simulink model "Y6_sim"  (R2024b)
settings: Solver=VariableStepAuto  StartTime=0.0  StopTime=580  RelTol=1e-3
values from neighbouring files (symbols this model uses):
  states0 = [42;0;0;0;0;0;0;0;0;0;0;0]    [Y6_params.m]
  timepoints = [0,30,55,80,105,130,165,190,215,240,265,300,325,350,375,400,435,460,485,510,535,570]    [Y6_params.m]
  waypoints = [42  ,42  ,42   ,42   ,42   ,42   ,31   ,31   ,31   ,31   ,31   ,20   ,20   ,20   ,20   ,20   ,9    ,9    ,9    ,9    ,9    ,9 ... (first row only)    [Y6_params.m]
libraries: shareduavrstlib x1, simulink x1, uavutilslib x1
settings Model: Creator=efymc10  LastModifiedBy=louis
settings SolverCC: ZeroCrossAlgorithm=Adaptive
settings DebuggingCC: IgnoredZcDiagnostic=none

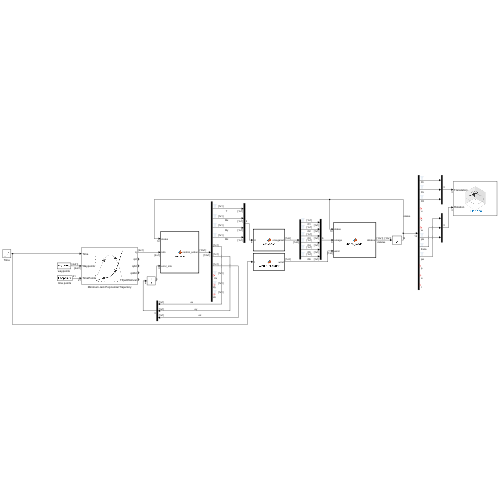
[thumbnail: Simulink's stored preview of the top-level diagram]
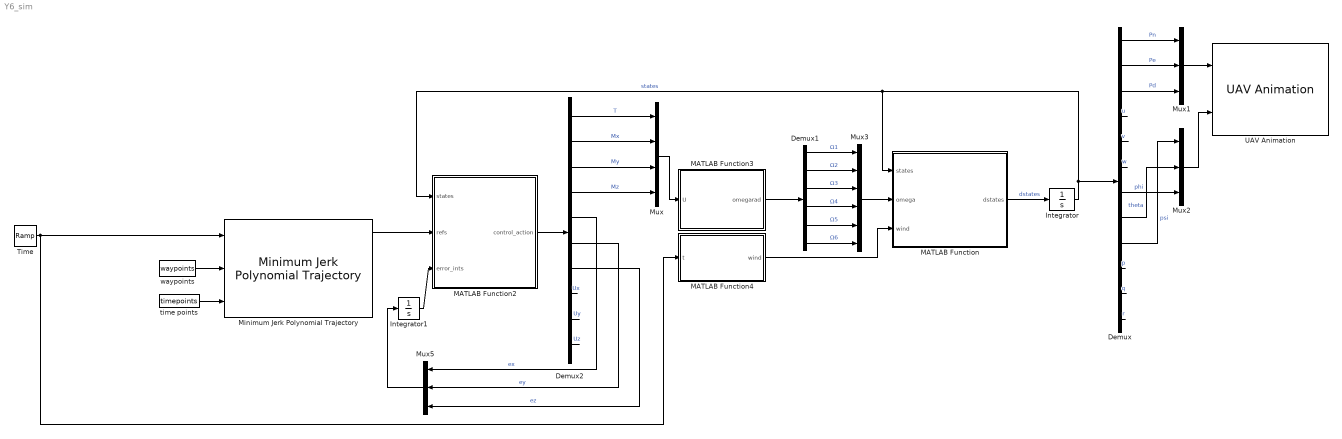
== system Y6_sim ==
  Demux : Demux  Outputs=12
  Demux1 : Demux  Outputs=6
  Demux2 : Demux  Outputs=10
  Integrator : Integrator  InitialCondition=states0
  Integrator1 : Integrator
  MATLAB Function : MATLAB Function  TreatAsAtomicUnit=on
  MATLAB Function2 : MATLAB Function  TreatAsAtomicUnit=on
  MATLAB Function3 : MATLAB Function  TreatAsAtomicUnit=on
  MATLAB Function4 : MATLAB Function  TreatAsAtomicUnit=on
  Minimum Jerk Polynomial Trajectory : shareduavrstlib/Minimum Jerk Polynomial Trajectory  ShowBCInputPort=off  ShowPolynomialCoefs=off  ShowStatusOutputPort=off  TimeAllocation=off  TimeWeight=100  MinSegmentTime=0.1  MaxSegmentTime=1  MaxIteration=1500  MaxTime=10  SimulateUsing=Interpreted execution
      settings: LibrarySourceBlock=uavalgslib/Minimum Jerk Polynomial Trajectory
  Mux : Mux
  Mux1 : Mux  Inputs=3
  Mux2 : Mux  Inputs=3
  Mux3 : Mux  Inputs=6
  Mux5 : Mux  Inputs=3
  Time : simulink/Sources/Ramp  slope=1  start=0  InitialOutput=0
  UAV Animation : uavutilslib/UAV Animation  NumUAV=1  DynamicUAVConfig=off  UAVType=Multirotor  UAVSize=1  UAVColor=[1 0 0]  UAVTrajectoryAlpha=1  InertialZDirection=Down  RotationFormat=Euler ZYX  DrawMarkers=off  SampleTime=0.01
  time points : Constant  Value=timepoints
  waypoints : Constant  Value=waypoints
  wires:
  Integrator/1 -> MATLAB Function2/1(states), MATLAB Function/1(states), Demux/1  "states"
  MATLAB Function/1(dstates) -> Integrator/1  "dstates"
  Demux/1 -> Mux1/1  "Pn"
  Demux/2 -> Mux1/2  "Pe"
  Demux/9 -> Mux2/1  "psi"
  Demux/7 -> Mux2/3  "phi"
  Demux/3 -> Mux1/3  "Pd"
  Demux/8 -> Mux2/2  "theta"
  Mux1/1 -> UAV Animation/1
  Mux2/1 -> UAV Animation/2
  time points/1 -> Minimum Jerk Polynomial Trajectory/3
  Minimum Jerk Polynomial Trajectory/1 -> MATLAB Function2/2(refs)
  Time/1 -> MATLAB Function4/1(t), Minimum Jerk Polynomial Trajectory/1
  MATLAB Function4/1(wind) -> MATLAB Function/3(wind)
  MATLAB Function2/1(control_action) -> Demux2/1
  Demux2/1 -> Mux/1  "T"
  Demux2/2 -> Mux/2  "Mx"
  Demux2/3 -> Mux/3  "My"
  Demux2/4 -> Mux/4  "Mz"
  Demux2/5 -> Mux5/1  "ex"
  Demux2/6 -> Mux5/2  "ey"
  Demux2/7 -> Mux5/3  "ez"
  Mux5/1 -> Integrator1/1
  Integrator1/1 -> MATLAB Function2/3(error_ints)
  Demux2/8 -> ?  "Ux"
  Demux2/9 -> ?  "Uy"
  Demux2/10 -> ?  "Uz"
  Demux/4 -> ?  "u"
  Demux/5 -> ?  "v"
  Demux/6 -> ?  "w"
  Demux/10 -> ?  "p"
  Demux/11 -> ?  "q"
  Demux/12 -> ?  "r"
  Demux1/1 -> Mux3/1  "Ω1"
  Demux1/2 -> Mux3/2  "Ω2"
  Demux1/3 -> Mux3/3  "Ω3"
  Demux1/4 -> Mux3/4  "Ω4"
  Demux1/5 -> Mux3/5  "Ω5"
  Demux1/6 -> Mux3/6  "Ω6"
  MATLAB Function3/1(omegarad) -> Demux1/1
  Mux3/1 -> MATLAB Function/2(omega)
  Mux/1 -> MATLAB Function3/1(U)
  waypoints/1 -> Minimum Jerk Polynomial Trajectory/2

== matlab function Y6_sim/MATLAB Function ==
  data: states input; dstates output; omega input; Y6 parameter; wind input
function dstates = drone_model(states, omega, Y6,wind)
    %obtaining relevant states from the last time step
    uvw = [states(4);states(5);states(6)];
    pqr = [states(10); states(11); states(12)];

    % DCM matrix
    phi=states(7); theta=states(8); psi=states(9);
    Cphi=cos(phi); Sphi=sin(phi);
    Ctheta=cos(theta); Stheta=sin(theta);
    Cpsi=cos(psi); Spsi=sin(psi);
    Rbv=[Ctheta*Cpsi, Sphi*Stheta*Cpsi-Cphi*Spsi, Cphi*Stheta*Cpsi+Sphi*Spsi;
         Ctheta*Spsi, Sphi*Stheta*Spsi+Cphi*Cpsi, Cphi*Stheta*Spsi-Sphi*Cpsi;
         -Stheta,     Sphi*Ctheta,                Cphi*Ctheta                ];

    %forces & moments
    % Extract motor speeds A-F is named according to document
    A = omega(1);  % Front-left top (CW)
    B = omega(2);  % Front-left bottom (CCW)
    C = omega(3);  % Front-right top (CW)
    D = omega(4);  % Front-right bottom (CCW)
    E = omega(5);  % Rear top (CCW)
    F = omega(6);  % Rear bottom (CW)
    
    % Calculate thrusts (F = k_T * ω^2)
    thrust_A = Y6.k_T * A^2;
    thrust_B = Y6.k_T * B^2;
    thrust_C = Y6.k_T * C^2;
    thrust_D = Y6.k_T * D^2;
    thrust_E = Y6.k_T * E^2;
    thrust_F = Y6.k_T * F^2;
    
    % Total thrust (sum of all motors)
    Uz = thrust_A + thrust_B + thrust_C + thrust_D + thrust_E + thrust_F;
    
    % Moments calculation
    % Roll (Mx): Difference between left and right front pairs
    Uphi = (Y6.L * sqrt(3)/2) * ((thrust_A + thrust_B) - (thrust_C + thrust_D));
    
    % Pitch (My): Front pairs vs rear pair
    Utheta = (Y6.L/2) * (thrust_A + thrust_B + thrust_C + thrust_D) - Y6.L * (thrust_E + thrust_F);
    
    % Yaw (Mz): Torque difference (CW motors: A, C, F; CCW motors: B, D, E)
    % Mz = k * (sum(CW) - sum(CCW)) = k * (A + C + F - B - D - E)
    Upsi = Y6.k * ( (A^2 + C^2 + F^2) - (B^2 + D^2 + E^2) );
    Fx=0; Fy=0; Fz=Uz;

    %simulate wind disturbance
    wind_x = wind(1);
    wind_y = wind(2);
    wind_force_body = [wind_x; wind_y; 0];  % Wind in body-frame XY plane (Z=0 for horizontal wind)
    wind_force_inertial = Rbv * wind_force_body;  % Convert to inertial frame

    Fp=[Fx;Fy;Fz]+wind_force_inertial;
    Fgi=[0;0;Y6.m*Y6.g];
    Fgb=Rbv'*Fgi;
    F=-Fp+Fgb;
    M=[Uphi;Utheta;Upsi];

    %kinematics eq(1)
    pned_dot=Rbv*uvw;

    %Dynamics eq(1)
    uvw_dot= cross(pqr,uvw)+F/Y6.m-0.25*uvw;

    %Phi Theta rotation eq(1)
    Ttheta=tan(theta);
    Rbe=[1, Sphi*Ttheta, Cphi*Ttheta;
         0, Cphi,        -Sphi;
         0, Sphi/Ctheta, Cphi/Ctheta];

    %kinematics eq(2)
    Euler_dot=Rbe*pqr;

    %inertia matrix
    J=[Y6.Ix, 0,       0;
       0,       Y6.Iy, 0;
       0,       0,       Y6.Iz];
    Jinv=inv(J);

    %dynamics eq(2)
    pqr_dot=Jinv*cross(pqr,J*pqr)+Jinv*M;

    dstates = [pned_dot; uvw_dot; Euler_dot; pqr_dot];
end

== matlab function Y6_sim/MATLAB Function2 ==
  data: states input; control_action output; refs input; error_ints input; Y6 parameter
function control_action = controller(states,refs,error_ints, Y6)
    %obtaining states
    pn = states(1); pe=states(2); pd=states(3);
    uvw = [states(4);states(5);states(6)];
    p=states(10); q=states(11); r=states(12);
    phi=states(7); theta=states(8); psi=states(9);

    %REFERENCES
    xref=refs(1); yref=refs(2); zref=refs(3); psiref=refs(4);
    
    %model and control coefficients
    m=Y6.m; g=Y6.g;
    kpx = 0.8; kix = 0.4 ; kdx = 0.45;
    kpy = 0.8; kiy = 0.4 ; kdy = 0.45;
    kpz = 8.0; kiz = 0.05; kdz = 5.6;
    
    kpphi = 3.0; kdphi = 0.4;
    kptheta = 3.0; kdtheta = 0.4;
    kppsi = 1.5; kdpsi = 20.8;

    %errors
    ex=xref-pn; ey=yref-pe; ez=zref-pd;
    ex_int=error_ints(1); ey_int=error_ints(2); ez_int=error_ints(3);

    %speeds in intertial frame
     % DCM matrix
    Cphi=cos(phi); Sphi=sin(phi);
    Ctheta=cos(theta); Stheta=sin(theta);
    Cpsi=cos(psi); Spsi=sin(psi);
    Rbv=[Ctheta*Cphi, Sphi*Stheta*Cpsi-Cphi*Spsi, Cphi*Stheta*Cpsi+Sphi*Spsi;
         Ctheta*Spsi, Sphi*Stheta*Spsi+Cphi*Cpsi, Cphi*Stheta*Spsi-Sphi*Cpsi;
         -Stheta,     Sphi*Ctheta,                Cphi*Ctheta                ];
    ifspd=Rbv*uvw;
    xspd=ifspd(1); yspd=ifspd(2); zspd=ifspd(3);

    %speed errors
    exdot=0-xspd; eydot=0-yspd; ezdot=0-zspd;

    %postition control
    Ux=kpx*ex+kdx*exdot+kix*ex_int; Uy=kpy*ey+kdy*eydot+kiy*ey_int; Uz=kpz*ez+kdz*ezdot+kiz*ez_int;

    T=m*(g-Uz);

    %attidude mapper
    thetaref=-(m*(Ux*cos(psi)+Uy*sin(psi)))/T;
    phiref=(m*(Uy*cos(psi)-Ux*sin(psi)))/T;

    %attitude errors
    ephi=phiref-phi; etheta=thetaref-theta; epsi=psiref-psi;
    ephidot=0-p; ethetadot=0-q; epsidot=0-r;

    %attitude control
    Mx=kpphi*ephi+kdphi*ephidot;
    My=kptheta*etheta+kdtheta*ethetadot;
    Mz=kppsi*epsi+kdpsi*epsidot;

    

control_action = [T;Mx;My;Mz;ex;ey;ez;Ux;Uy;Uz];
end

== matlab function Y6_sim/MATLAB Function3 ==
  data: omegarad output; Y6 parameter; U input
function omegarad = converter(Y6, U)
    %assigning forces and moments
    F_total = U(1); Mx = U(2); My = U(3); Mz = U(4);
    %assigning params
    L = Y6.L; k_t = Y6.k_T; k = Y6.k;
    
    % Solve for summed/differential thrusts
    T_AB = max((F_total/3 + 2*My/(3*L)) + Mx/(L*sqrt(3)),0);
    T_CD = max((F_total/3 + 2*My/(3*L)) - Mx/(L*sqrt(3)),0);
    T_E = max((F_total/6 - 4*My/(6*L)) - Mz/(2*k), 0);
    T_F = max((F_total/6 - 4*My/(6*L)) + Mz/(2*k), 0);
    
    % Distribute thrusts to individual motors
    A = T_AB/2; B = T_AB/2;  % Equal split for AB pair
    C = T_CD/2; D = T_CD/2;  % Equal split for CD pair
    E = T_E; F = T_F;        % Independent rear motors
    
    % Convert to rad/s
    thrusts = [A, B, C, D, E, F];
    omegarad = sqrt(max(thrusts, 0) / k_t);
end

== matlab function Y6_sim/MATLAB Function4 ==
  data: t input; wind output; max_wind parameter
function wind = Wind_Generator(t,max_wind)
% Input: 
%   t - Simulation time (from Ramp block)
% Output:
%   wind_x, wind_y - Wind forces in body X/Y axes (N)

% --- Wind Profile Parameters ---
wind_start_time = 3.0;   % Start wind at t=5s
wind_steady_time = 10.0; % Reach full strength at t=30s

% --- Generate wind ---
if t < wind_start_time
    wind_x = 0;  % No wind initially
    wind_y = 0;
elseif t < wind_steady_time
    % Ramp up wind linearly (e.g., gust building)
    wind_x = max_wind * (t - wind_start_time) / (wind_steady_time - wind_start_time);
    wind_y = 0;
else
    % Steady-state wind
    wind_x = max_wind;
    wind_y = 0;
end
    wind=[wind_x,wind_y];
end
